simulink model "test"  (R2018b)
settings: Solver=VariableStepAuto  StartTime=0.0  StopTime=10.0  RelTol=1e-3
settings Model: Creator=willr  LastModifiedBy=willr

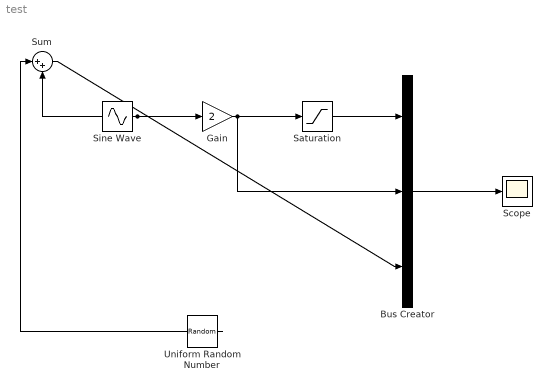
== system test ==
  Bus Creator : BusCreator  Inputs=3
  Gain : Gain  Gain=2
  Saturation : Saturate
  Scope : Scope
  Sine Wave : Sin  SampleTime=0
  Sum : Sum  Inputs=|++
  Uniform Random Number : UniformRandomNumber  SampleTime=0.1
  wires:
  Sine Wave/1 -> Gain/1, Sum/2
  Gain/1 -> Saturation/1, Bus Creator/2
  Saturation/1 -> Bus Creator/1
  Bus Creator/1 -> Scope/1
  Uniform Random Number/1 -> Sum/1
  Sum/1 -> Bus Creator/3
